simulink model "ControlledGrid"  (R2015b)
settings: Solver=ode1  StartTime=0.0  StopTime=10  FixedStep=Ts  RelTol=1e-3
InitFcn:
  | ControlInit();
values from neighbouring files (symbols this model uses):
  Fnom = 50    [ControlInit.m]
  Grid_F = Fnom    (= 50)    [ControlInit.m]
  Grid_V = 400e3    (= 400000)    [ControlInit.m]
  Rad2Deg = 180/pi    (= 57.2956455309)    [ControlInit.m]
libraries: powerlib x16, powerlib_meascontrol x3, simulink x2
settings Model: Creator=Emilio  LastModifiedBy=Emilio

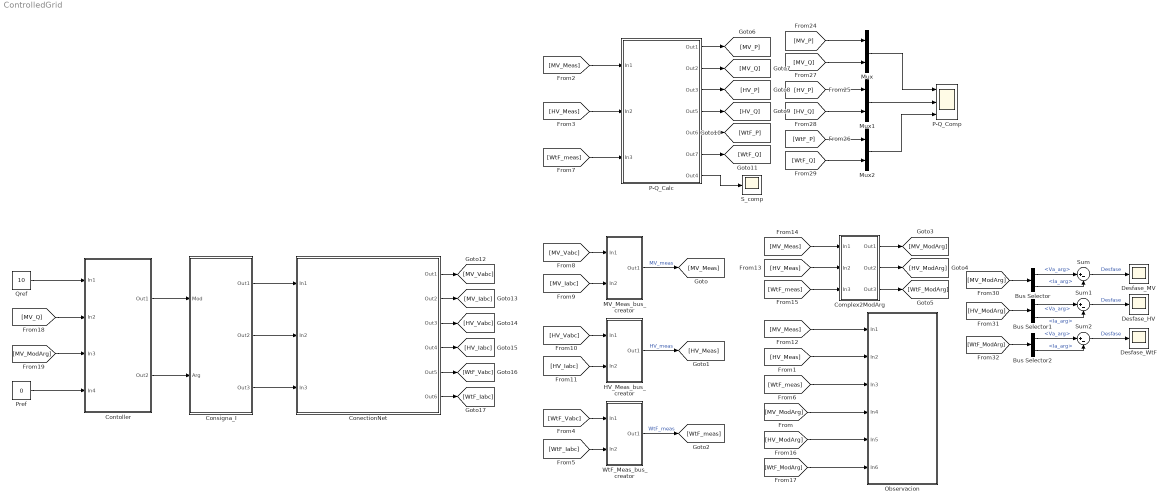
== system ControlledGrid ==
  Bus Selector : BusSelector  OutputSignals=V_ModArg.Va_arg,I_ModArg.Ia_arg
  Bus Selector1 : BusSelector  OutputSignals=V_ModArg.Va_arg,I_ModArg.Ia_arg
  Bus Selector2 : BusSelector  OutputSignals=V_ModArg.Va_arg,I_ModArg.Ia_arg
  Complex2ModArg : Subsystem
  ConectionNet : Subsystem
  Consigna_I : Subsystem
  Contoller : Subsystem
  Desfase_HV : Scope
  Desfase_MV : Scope
  Desfase_WtF : Scope
  HV_Meas_bus_creator : Subsystem
  MV_Meas_bus_creator : Subsystem
  Mux : Mux  Inputs=2
  Mux1 : Mux  Inputs=2
  Mux2 : Mux  Inputs=2
  Observacion : Subsystem
  P-Q_Calc : Subsystem
  P-Q_Comp : Scope  NumInputPorts=3
  Pref : Constant  Value=0
  Qref : Constant  Value=10
  S_comp : Scope
  Sum : Sum  Inputs=|+-
  Sum1 : Sum  Inputs=|+-
  Sum2 : Sum  Inputs=|+-
  WtF_Meas_bus_creator : Subsystem
  wires:
  [MV_Meas] -> P-Q_Calc/1(In1)
  [HV_Meas] -> P-Q_Calc/2(In2)
  P-Q_Calc/7(Out4) -> S_comp/1
  [MV_Vabc] -> MV_Meas_bus_creator/1(In1)
  [MV_Iabc] -> MV_Meas_bus_creator/2(In2)
  MV_Meas_bus_creator/1(Out1) -> [MV_Meas]  "MV_meas"
  [HV_Vabc] -> HV_Meas_bus_creator/1(In1)
  [HV_Iabc] -> HV_Meas_bus_creator/2(In2)
  HV_Meas_bus_creator/1(Out1) -> [HV_Meas]  "HV_meas"
  [WtF_Vabc] -> WtF_Meas_bus_creator/1(In1)
  [WtF_Iabc] -> WtF_Meas_bus_creator/2(In2)
  WtF_Meas_bus_creator/1(Out1) -> [WtF_meas]  "WtF_meas"
  [WtF_meas] -> P-Q_Calc/3(In3)
  [MV_Meas] -> Observacion/1(In1)
  [HV_Meas] -> Observacion/2(In2)
  [WtF_meas] -> Observacion/3(In3)
  [MV_ModArg] -> Observacion/4(In4)
  [HV_ModArg] -> Observacion/5(In5)
  [WtF_ModArg] -> Observacion/6(In6)
  P-Q_Calc/1(Out1) -> [MV_P]
  P-Q_Calc/2(Out2) -> [MV_Q]
  P-Q_Calc/3(Out3) -> [HV_P]
  P-Q_Calc/4(Out5) -> [HV_Q]
  P-Q_Calc/5(Out6) -> [WtF_P]
  P-Q_Calc/6(Out7) -> [WtF_Q]
  ConectionNet/1(Out1) -> [MV_Vabc]
  ConectionNet/2(Out2) -> [MV_Iabc]
  ConectionNet/3(Out3) -> [HV_Vabc]
  ConectionNet/4(Out4) -> [HV_Iabc]
  ConectionNet/5(Out5) -> [WtF_Vabc]
  ConectionNet/6(Out6) -> [WtF_Iabc]
  Consigna_I/1(Out1) -> ConectionNet/1(In1)
  Consigna_I/2(Out2) -> ConectionNet/2(In2)
  Consigna_I/3(Out3) -> ConectionNet/3(In3)
  [MV_Meas] -> Complex2ModArg/1(In1)
  [HV_Meas] -> Complex2ModArg/2(In2)
  [WtF_meas] -> Complex2ModArg/3(In3)
  Complex2ModArg/1(Out1) -> [MV_ModArg]
  Complex2ModArg/2(Out2) -> [HV_ModArg]
  Complex2ModArg/3(Out3) -> [WtF_ModArg]
  [MV_P] -> Mux/1
  [MV_Q] -> Mux/2
  [HV_Q] -> Mux1/2
  [HV_P] -> Mux1/1
  [WtF_P] -> Mux2/1
  [WtF_Q] -> Mux2/2
  Mux/1 -> P-Q_Comp/1
  Mux1/1 -> P-Q_Comp/2
  Mux2/1 -> P-Q_Comp/3
  [MV_ModArg] -> Bus Selector/1
  Bus Selector/1 -> Sum/1  "<Va_arg>"
  Bus Selector/2 -> Sum/2  "<Ia_arg>"
  Sum/1 -> Desfase_MV/1  "Desfase"
  [HV_ModArg] -> Bus Selector1/1
  Bus Selector1/1 -> Sum1/1  "<Va_arg>"
  Bus Selector1/2 -> Sum1/2  "<Ia_arg>"
  Sum1/1 -> Desfase_HV/1  "Desfase"
  Bus Selector2/1 -> Sum2/1  "<Va_arg>"
  Bus Selector2/2 -> Sum2/2  "<Ia_arg>"
  Sum2/1 -> Desfase_WtF/1  "Desfase"
  [WtF_ModArg] -> Bus Selector2/1
  Qref/1 -> Contoller/1(In1)
  [MV_Q] -> Contoller/2(In2)
  [MV_ModArg] -> Contoller/3(In3)
  Contoller/1(Out1) -> Consigna_I/1(Mod)
  Pref/1 -> Contoller/4(In4)
  Contoller/2(Out2) -> Consigna_I/2(Arg)

== system ControlledGrid/Complex2ModArg ==
  In1 : Inport
  In2 : Inport  Port=2
  In3 : Inport  Port=3
  Bus Creator1 : BusCreator  Inputs=2
  Bus Creator2 : BusCreator  Inputs=2
  Bus Creator3 : BusCreator  Inputs=2
  Bus Selector3 : BusSelector  OutputSignals=V_meas.Va,V_meas.Vb,V_meas.Vc,I_meas.Ia,I_meas.Ib,I_meas.Ic
  Bus Selector4 : BusSelector  OutputSignals=V_meas.Va,V_meas.Vb,V_meas.Vc,I_meas.Ia,I_meas.Ib,I_meas.Ic
  Bus Selector5 : BusSelector  OutputSignals=V_meas.Va,V_meas.Vb,V_meas.Vc,I_meas.Ia,I_meas.Ib,I_meas.Ic
  HV_mod&arg : Subsystem
  MV_mod&arg : Subsystem
  WtF_mod&arg : Subsystem
  Out1 : Outport
  Out2 : Outport  Port=2
  Out3 : Outport  Port=3
  wires:
  Bus Selector4/1 -> WtF_mod&arg/1(In1)  "<Va>"
  Bus Selector3/1 -> HV_mod&arg/1(In1)  "<Va>"
  Bus Selector3/2 -> HV_mod&arg/2(In2)  "<Vb>"
  Bus Selector3/3 -> HV_mod&arg/3(In3)  "<Vc>"
  Bus Selector3/4 -> HV_mod&arg/4(In4)  "<Ia>"
  Bus Selector3/6 -> HV_mod&arg/6(In6)  "<Ic>"
  HV_mod&arg/1(Out1) -> Bus Creator3/1
  In2/1 -> Bus Selector3/1
  HV_mod&arg/2(Out2) -> Bus Creator3/2
  In3/1 -> Bus Selector4/1
  Bus Selector3/5 -> HV_mod&arg/5(In5)  "<Ib>"
  Bus Selector4/6 -> WtF_mod&arg/6(In6)  "<Ic>"
  MV_mod&arg/1(Out1) -> Bus Creator2/1
  Bus Selector5/3 -> MV_mod&arg/3(In3)  "<Vc>"
  Bus Selector4/3 -> WtF_mod&arg/3(In3)  "<Vc>"
  Bus Selector4/2 -> WtF_mod&arg/2(In2)  "<Vb>"
  Bus Selector4/5 -> WtF_mod&arg/5(In5)  "<Ib>"
  Bus Creator3/1 -> Out2/1  "HV_ModArg"
  Bus Selector5/1 -> MV_mod&arg/1(In1)  "<Va>"
  Bus Selector5/6 -> MV_mod&arg/6(In6)  "<Ic>"
  Bus Selector5/5 -> MV_mod&arg/5(In5)  "<Ib>"
  Bus Creator2/1 -> Out1/1  "MV_ModArg"
  Bus Selector5/2 -> MV_mod&arg/2(In2)  "<Vb>"
  Bus Creator1/1 -> Out3/1  "WtF_ModArg"
  WtF_mod&arg/1(Out1) -> Bus Creator1/1
  WtF_mod&arg/2(Out2) -> Bus Creator1/2
  MV_mod&arg/2(Out2) -> Bus Creator2/2
  Bus Selector4/4 -> WtF_mod&arg/4(In4)  "<Ia>"
  Bus Selector5/4 -> MV_mod&arg/4(In4)  "<Ia>"
  In1/1 -> Bus Selector5/1

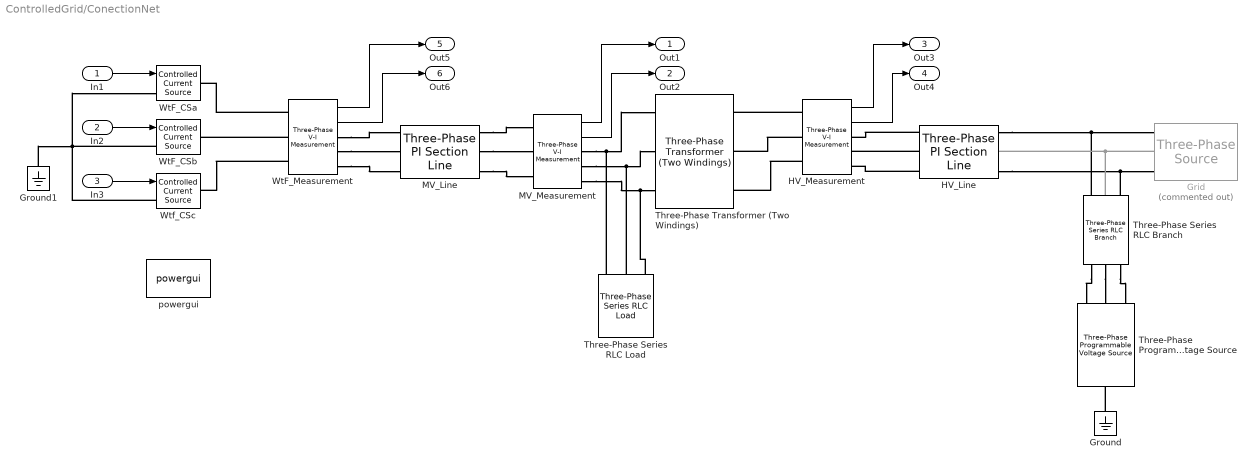
== system ControlledGrid/ConectionNet ==
  In1 : Inport
  In2 : Inport  Port=2
  In3 : Inport  Port=3
  Grid : powerlib/Electrical Sources/Three-Phase Source  Commented=on  InternalConnection=Yg  VoltagePhases=off  Voltage=Grid_V  PhaseAngle=0  Voltage_phases=[25e3 25e3 25e3]/sqrt(3)  PhaseAngles_phases=[0 -120 +120]  Frequency=Grid_F  NonIdealSource=on  SpecifyImpedance=off  Resistance=0.8929  Inductance=16.58e-3  ShortCircuitLevel=100e6  BaseVoltage=25e3  XRratio=7  BusType=PQ  Pref=10e3  Qref=0  Prefabc=[10e3, 10e3, 10e3]  Qrefabc=[0, 0, 0]  Qmin=-inf  Qmax=inf
  Ground : powerlib/Elements/Ground  LConnTagsString=a
  Ground1 : powerlib/Elements/Ground  LConnTagsString=a
  HV_Line : powerlib/Elements/Three-Phase PI Section Line  LConnTagsString=a|b|c  RConnTagsString=A|B|C  Frequency=50  Resistances=[ 0.01273 0.3864]  Inductances="[ 0.9337e-3  4.1264e-3]"  Capacitances=[12.74e-9 7.751e-9]  Length=100
  HV_Measurement : powerlib/Measurements/Three-Phase V-I Measurement  VoltageMeasurement=phase-to-ground  SetLabelV=off  LabelV=HV_Vabc  Vpu=off  VpuLL=off  CurrentMeasurement=yes  SetLabelI=off  LabelI=HV_Iabc  Ipu=off  Pbase=100e6  Vbase=500e3  OutputType=Complex  PhasorSimulation=on  PSBequivalent=0
  MV_Line : powerlib/Elements/Three-Phase PI Section Line  LConnTagsString=a|b|c  RConnTagsString=A|B|C  Frequency=50  Resistances=[ 0.01273 0.3864]  Inductances="[ 0.9337e-3  4.1264e-3]"  Capacitances="[ 0.9337e-3  4.1264e-3]"  Length=20
  MV_Measurement : powerlib/Measurements/Three-Phase V-I Measurement  VoltageMeasurement=phase-to-ground  SetLabelV=off  LabelV=MV_Vabc  Vpu=off  VpuLL=off  CurrentMeasurement=yes  SetLabelI=off  LabelI=MV_Iabc  Ipu=off  Pbase=100e6  Vbase=500e3  OutputType=Complex  PhasorSimulation=on  PSBequivalent=0
  Three-Phase Programmable Voltage Source : powerlib/Electrical Sources/Three-Phase Programmable Voltage Source  PositiveSequence="[Grid_V  0 Grid_F]"  VariationEntity=Amplitude  VariationType=Modulation  VariationTypeAlt=Step  VariationStep=0.5  VariationRate=10  VariationMagnitude=0  VariationFrequency=0.10  VariationTiming=[0 10]  VariationPhaseA=off  Amplitudes=[1 0.8 1.2 1.0]  TimeValues=[0 0.1 0.15 0.2]  HarmonicGeneration=off  HarmonicA=[3 0.2 -25 0]  HarmonicB=[2 0.15 35 2]  Timing="[0.05  3]"  BusType=PQ  Pref=0  Qref=0  Qmin=-inf  Qmax=inf
  Three-Phase Series RLC Branch : powerlib/Elements/Three-Phase Series RLC Branch  LConnTagsString=A|B|C  RConnTagsString=A|B|C  BranchType=RL  Resistance=1  Inductance=16.58e-3  Capacitance=0  Measurements=None
  Three-Phase Series RLC Load : powerlib/Elements/Three-Phase Series RLC Load  LConnTagsString=A|B|C  Configuration=Y (grounded)  NominalVoltage=1000  Vabc=[1e3 1e3 1e3]  Vabcp=[1e3 1e3 1e3]  NominalFrequency=60  UnbalancedPower=off  ActivePower=1  InductivePower=0  CapacitivePower=150e6  Pabc=[10e3 9e3 11e3]  QLabc=[100 90 110]  QCabc=[100 90 110]  Pabcp=[10e3 9e3 11e3]  QLabcp=[100 90 110]  QCabcp=[100 90 110]  Measurements=None  LoadType=constant Z
  Three-Phase Transformer (Two Windings) : powerlib/Elements/Three-Phase Transformer (Two Windings)  Winding1Connection=Yg  Winding2Connection=Yg  CoreType=Three single-phase transformers  SetSaturation=off  Hysteresis=off  DataFile='hysteresis'  SetInitialFlux=off  Measurements=None  UNITS=SI  NominalPower=[ 100e3 , 50 ]  Winding1=[22000 9.68 0.030812]  Winding2=[4e+05 3200 10.186]  Rm=2.42e+06  Lm=7703.1  L0=7.7033  Saturation=[0 0;0.0089072 68.613;3.7113 86.91]  InitialFluxes=[45.742 -45.742 40.024]  MoreParameters=off  BreakLoop=off  DataType=on  TransfoNumber=1
  WtF_CSa : powerlib/Electrical Sources/Controlled Current Source  Initialize=on  Source_Type=AC  Amplitude=12.9  Phase=0  Frequency=Fnom  Measurements=None
  WtF_CSb : powerlib/Electrical Sources/Controlled Current Source  Initialize=on  Source_Type=AC  Amplitude=12.9  Phase=120  Frequency=Fnom  Measurements=None
  WtF_Measurement : powerlib/Measurements/Three-Phase V-I Measurement  VoltageMeasurement=phase-to-ground  SetLabelV=off  LabelV=WtF_Vabc  Vpu=off  VpuLL=off  CurrentMeasurement=yes  SetLabelI=off  LabelI=WtF_Iabc  Ipu=off  Pbase=100e6  Vbase=500e3  OutputType=Complex  PhasorSimulation=on  PSBequivalent=0
  Wtf_CSc : powerlib/Electrical Sources/Controlled Current Source  Initialize=on  Source_Type=AC  Amplitude=12.9  Phase=-120  Frequency=Fnom  Measurements=None
  powergui : powerlib/powergui  Priority=1  SimulationMode=Phasor  SolverType=Tustin/Backward Euler (TBE)  SampleTime=50e-6  frequency=Fnom  SPID=off  DisableSnubberDevices=off  DisableRonSwitches=off  DisableVfSwitches=off  SwTol=0  DisplayEquations=off  Interpol=off  ExternalGateDelay=off  methode=off  Ts=10  FunctionMessages=off  echomessages=off  HookPort=off  EnableUseOfTLC=off  x0status=blocks  frequencyindice=50  Pbase=100e6  ErrMax=1e-4  Iterations=50  UnitsV=V  UnitsW=W  buscounter=0  RestoreLinks=warning  ResistiveCurrentMeasurement=off  Frange=[0:2:500]  Ylog=off  Xlog=on  ShowGrid=off  save=off  variable=ZData  structure=0  ZoomFFT=off  StartTime=0.0  cycles=1  DisplayStyle=1  fundamental=60  FreqAxis=off  MaxFrequency=1000  frequencyindicesteady=1  RmsSteady=1  display=off
  Out1 : Outport
  Out2 : Outport  Port=2
  Out3 : Outport  Port=3
  Out4 : Outport  Port=4
  Out5 : Outport  Port=5
  Out6 : Outport  Port=6
  wires:
  In1/1 -> WtF_CSa/1
  In2/1 -> WtF_CSb/1
  In3/1 -> Wtf_CSc/1
  MV_Measurement/1 -> Out1/1
  HV_Measurement/1 -> Out3/1
  HV_Measurement/2 -> Out4/1
  MV_Measurement/2 -> Out2/1
  WtF_Measurement/1 -> Out5/1
  WtF_Measurement/2 -> Out6/1
  connections:
  HV_Line/LConn2 -- HV_Measurement/RConn2
  HV_Measurement/LConn2 -- Three-Phase Transformer (Two Windings)/RConn2
  Three-Phase Series RLC Branch/LConn3 -- HV_Line/RConn3 -- Grid/RConn1
  HV_Line/RConn1 -- Three-Phase Series RLC Branch/LConn1 -- Grid/RConn3
  Grid/RConn2 -- Three-Phase Series RLC Branch/LConn2 -- HV_Line/RConn2
  HV_Measurement/LConn1 -- Three-Phase Transformer (Two Windings)/RConn1
  HV_Measurement/LConn3 -- Three-Phase Transformer (Two Windings)/RConn3
  MV_Measurement/RConn2 -- Three-Phase Series RLC Load/LConn2 -- Three-Phase Transformer (Two Windings)/LConn2
  MV_Measurement/RConn3 -- Three-Phase Series RLC Load/LConn3 -- Three-Phase Transformer (Two Windings)/LConn3
  MV_Measurement/RConn1 -- Three-Phase Transformer (Two Windings)/LConn1 -- Three-Phase Series RLC Load/LConn1
  HV_Line/LConn1 -- HV_Measurement/RConn1
  MV_Line/RConn1 -- MV_Measurement/LConn1
  MV_Line/RConn3 -- MV_Measurement/LConn3
  WtF_Measurement/LConn3 -- Wtf_CSc/RConn1
  WtF_Measurement/LConn1 -- WtF_CSa/RConn1
  MV_Line/RConn2 -- MV_Measurement/LConn2
  WtF_Measurement/LConn2 -- WtF_CSb/RConn1
  Ground/LConn1 -- Three-Phase Programmable Voltage Source/LConn1
  Three-Phase Series RLC Branch/RConn3 -- Three-Phase Programmable Voltage Source/RConn3
  Three-Phase Series RLC Branch/RConn1 -- Three-Phase Programmable Voltage Source/RConn1
  Three-Phase Series RLC Branch/RConn2 -- Three-Phase Programmable Voltage Source/RConn2
  WtF_Measurement/RConn3 -- MV_Line/LConn3
  WtF_Measurement/RConn2 -- MV_Line/LConn2
  WtF_Measurement/RConn1 -- MV_Line/LConn1
  HV_Line/LConn3 -- HV_Measurement/RConn3
  Wtf_CSc/LConn1 -- WtF_CSa/LConn1 -- Ground1/LConn1 -- WtF_CSb/LConn1

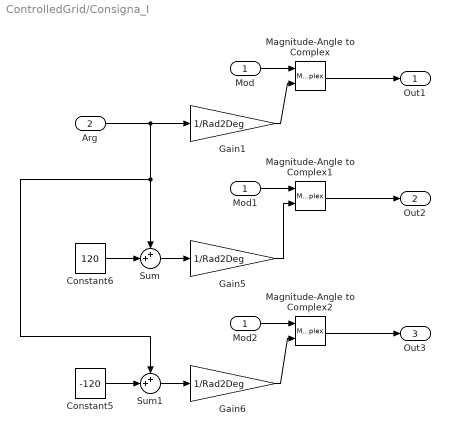
== system ControlledGrid/Consigna_I ==
  Mod : Inport
  Arg : Inport  Port=2
  Constant5 : Constant  Value=-120
  Constant6 : Constant  Value=120
  Gain1 : Gain  Gain=1/Rad2Deg
  Gain5 : Gain  Gain=1/Rad2Deg
  Gain6 : Gain  Gain=1/Rad2Deg
  Magnitude-Angle to Complex : MagnitudeAngleToComplex
  Magnitude-Angle to Complex1 : MagnitudeAngleToComplex
  Magnitude-Angle to Complex2 : MagnitudeAngleToComplex
  Mod1 : InportShadow
  Mod2 : InportShadow
  Sum : Sum  Inputs=++|
  Sum1 : Sum  Inputs=++|
  Out1 : Outport
  Out2 : Outport  Port=2
  Out3 : Outport  Port=3
  wires:
  Magnitude-Angle to Complex/1 -> Out1/1
  Magnitude-Angle to Complex1/1 -> Out2/1
  Magnitude-Angle to Complex2/1 -> Out3/1
  Gain5/1 -> Magnitude-Angle to Complex1/2
  Gain6/1 -> Magnitude-Angle to Complex2/2
  Mod2/1 -> Magnitude-Angle to Complex2/1
  Mod1/1 -> Magnitude-Angle to Complex1/1
  Mod/1 -> Magnitude-Angle to Complex/1
  Arg/1 -> Gain1/1, Sum/1, Sum1/1
  Sum1/1 -> Gain6/1
  Constant5/1 -> Sum1/2
  Sum/1 -> Gain5/1
  Constant6/1 -> Sum/2
  Gain1/1 -> Magnitude-Angle to Complex/2

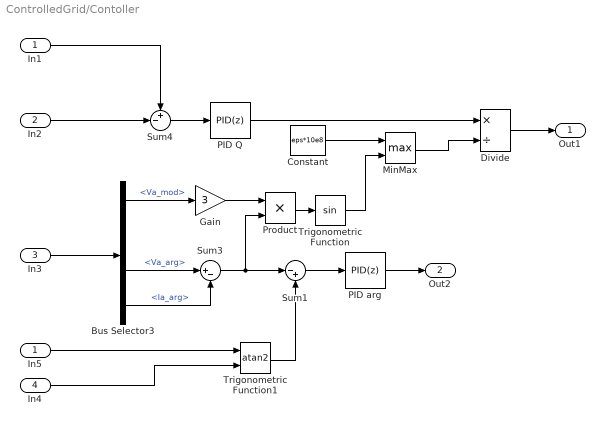
== system ControlledGrid/Contoller ==
  In1 : Inport
  In2 : Inport  Port=2
  In3 : Inport  Port=3
  In4 : Inport  Port=4
  " PID arg" : simulink/Continuous/PID Controller  Controller=PID  TimeDomain=Discrete-time  SampleTime=-1  IntegratorMethod=Forward Euler  FilterMethod=Forward Euler  Form=Parallel  UseFilter=on  ControllerParametersSource=internal  P=1  I=1  D=0  N=100  InitialConditionSource=internal  InitialConditionForIntegrator=0  InitialConditionForFilter=0  ExternalReset=none  LimitOutput=off  UpperSaturationLimit=inf  LowerSaturationLimit=-inf  LinearizeAsGain=off  AntiWindupMode=none  Kb=1  TrackingMode=off  Kt=1  PParamMin=[]  PParamMax=[]  IParamMin=[]  IParamMax=[]  DParamMin=[]  DParamMax=[]  NParamMin=[]  NParamMax=[]  KbParamMin=[]  KbParamMax=[]  KtParamMin=[]  KtParamMax=[]  POutMin=[]  POutMax=[]  IOutMin=[]  IOutMax=[]  DOutMin=[]  DOutMax=[]  NOutMin=[]  NOutMax=[]  KbOutMin=[]  KbOutMax=[]  KtOutMin=[]  KtOutMax=[]  IntegratorOutMin=[]  IntegratorOutMax=[]  FilterOutMin=[]  FilterOutMax=[]  SumOutMin=[]  SumOutMax=[]  SumI1OutMin=[]  SumI1OutMax=[]  SumI2OutMin=[]  SumI2OutMax=[]  SumI3OutMin=[]  SumI3OutMax=[]  SumDOutMin=[]  SumDOutMax=[]  SaturationOutMin=[]  SaturationOutMax=[]  IntegratorContinuousStateAttributes=''  IntegratorStateMustResolveToSignalObject=off  IntegratorRTWStateStorageClass=Auto  FilterContinuousStateAttributes=''  FilterStateMustResolveToSignalObject=off  FilterRTWStateStorageClass=Auto  DifferentiatorICPrevScaledInput=0  DifferentiatorOutMin=[]  DifferentiatorOutMax=[]
  Bus Selector3 : BusSelector  OutputSignals=V_ModArg.Va_mod,I_ModArg.Ia_mod,V_ModArg.Va_arg,I_ModArg.Ia_arg
  Constant : Constant  Value=eps*10e8  OutDataTypeStr=double
  Divide : Product  Inputs=*/
  Gain : Gain  Gain=3
  In5 : InportShadow
  MinMax : MinMax  Function=max  Inputs=2
  PID Q : simulink/Continuous/PID Controller  Controller=PID  TimeDomain=Discrete-time  SampleTime=-1  IntegratorMethod=Forward Euler  FilterMethod=Forward Euler  Form=Parallel  UseFilter=on  ControllerParametersSource=internal  P=1  I=1  D=0  N=100  InitialConditionSource=internal  InitialConditionForIntegrator=0  InitialConditionForFilter=0  ExternalReset=none  LimitOutput=off  UpperSaturationLimit=inf  LowerSaturationLimit=-inf  LinearizeAsGain=off  AntiWindupMode=none  Kb=1  TrackingMode=off  Kt=1  PParamMin=[]  PParamMax=[]  IParamMin=[]  IParamMax=[]  DParamMin=[]  DParamMax=[]  NParamMin=[]  NParamMax=[]  KbParamMin=[]  KbParamMax=[]  KtParamMin=[]  KtParamMax=[]  POutMin=[]  POutMax=[]  IOutMin=[]  IOutMax=[]  DOutMin=[]  DOutMax=[]  NOutMin=[]  NOutMax=[]  KbOutMin=[]  KbOutMax=[]  KtOutMin=[]  KtOutMax=[]  IntegratorOutMin=[]  IntegratorOutMax=[]  FilterOutMin=[]  FilterOutMax=[]  SumOutMin=[]  SumOutMax=[]  SumI1OutMin=[]  SumI1OutMax=[]  SumI2OutMin=[]  SumI2OutMax=[]  SumI3OutMin=[]  SumI3OutMax=[]  SumDOutMin=[]  SumDOutMax=[]  SaturationOutMin=[]  SaturationOutMax=[]  IntegratorContinuousStateAttributes=''  IntegratorStateMustResolveToSignalObject=off  IntegratorRTWStateStorageClass=Auto  FilterContinuousStateAttributes=''  FilterStateMustResolveToSignalObject=off  FilterRTWStateStorageClass=Auto  DifferentiatorICPrevScaledInput=0  DifferentiatorOutMin=[]  DifferentiatorOutMax=[]
  Product : Product
  Sum1 : Sum  Inputs=|-+
  Sum3 : Sum  Inputs=|+-
  Sum4 : Sum  Inputs=+-|
  Trigonometric Function : Trigonometry
  Trigonometric Function1 : Trigonometry  Operator=atan2
  Out1 : Outport
  Out2 : Outport  Port=2
  wires:
  Gain/1 -> Product/1
  Bus Selector3/4 -> Sum3/2  "<Ia_arg>"
  In3/1 -> Bus Selector3/1
  Sum3/1 -> Sum1/1, Product/2
  Bus Selector3/1 -> Gain/1  "<Va_mod>"
  Bus Selector3/3 -> Sum3/1  "<Va_arg>"
  In2/1 -> Sum4/2
  In1/1 -> Sum4/1
  Sum4/1 -> PID Q/1
  PID Q/1 -> Divide/1
  Divide/1 -> Out1/1
  Product/1 -> Trigonometric Function/1
  " PID arg"/1 -> Out2/1
  Sum1/1 -> " PID arg"/1
  In5/1 -> Trigonometric Function1/1
  In4/1 -> Trigonometric Function1/2
  Trigonometric Function1/1 -> Sum1/2
  MinMax/1 -> Divide/2
  Trigonometric Function/1 -> MinMax/2
  Constant/1 -> MinMax/1

== system ControlledGrid/HV_Meas_bus_creator ==
  In1 : Inport
  In2 : Inport  Port=2
  " " : ComplexToRealImag
  " 1" : ComplexToRealImag
  Bus Creator : BusCreator  Inputs=2
  Bus Creator1 : BusCreator  Inputs=6
  Bus Creator2 : BusCreator  Inputs=6
  Demux4 : Demux  Outputs=3
  Demux5 : Demux  Outputs=3
  Out1 : Outport  OutDataTypeStr=Bus: HV_meas
  wires:
  " "/1 -> Bus Creator2/3  "Ia_real"
  In1/1 -> Demux4/1, Bus Creator1/1  "Vabc"
  In2/1 -> Demux5/1, Bus Creator2/1  "Iabc"
  " 1"/2 -> Bus Creator1/4  "Va_img"
  Demux4/1 -> " 1"/1, Bus Creator1/2  "Va"
  Demux4/2 -> Bus Creator1/5  "Vb"
  Demux5/3 -> Bus Creator2/6  "Ic"
  " "/2 -> Bus Creator2/4  "Ia_img"
  Demux5/2 -> Bus Creator2/5  "Ib"
  Bus Creator/1 -> Out1/1
  " 1"/1 -> Bus Creator1/3  "Va_real"
  Demux5/1 -> Bus Creator2/2, " "/1  "Ia"
  Bus Creator2/1 -> Bus Creator/2  "I_meas"
  Bus Creator1/1 -> Bus Creator/1  "V_meas"
  Demux4/3 -> Bus Creator1/6  "Vc"

== system ControlledGrid/MV_Meas_bus_creator ==
  note: Creacion de los buses de medidas de los parametros de la red
  In1 : Inport
  In2 : Inport  Port=2
  " " : ComplexToRealImag
  "  " : ComplexToRealImag
  Bus Creator : BusCreator  Inputs=2
  Bus Creator1 : BusCreator  Inputs=6
  Bus Creator2 : BusCreator  Inputs=6
  Demux4 : Demux  Outputs=3
  Demux5 : Demux  Outputs=3
  Out1 : Outport  OutDataTypeStr=Bus: MV_meas
  wires:
  Demux4/3 -> Bus Creator1/6  "Vc"
  Bus Creator1/1 -> Bus Creator/1  "V_meas"
  Bus Creator2/1 -> Bus Creator/2  "I_meas"
  Demux5/1 -> " "/1, Bus Creator2/2  "Ia"
  "  "/1 -> Bus Creator1/3  "Va_real"
  Bus Creator/1 -> Out1/1
  Demux5/2 -> Bus Creator2/5  "Ib"
  " "/2 -> Bus Creator2/4  "Ia_img"
  Demux5/3 -> Bus Creator2/6  "Ic"
  Demux4/2 -> Bus Creator1/5  "Vb"
  Demux4/1 -> Bus Creator1/2, "  "/1  "Va"
  "  "/2 -> Bus Creator1/4  "Va_img"
  In2/1 -> Bus Creator2/1, Demux5/1  "Iabc"
  In1/1 -> Bus Creator1/1, Demux4/1  "Vabc"
  " "/1 -> Bus Creator2/3  "Ia_real"

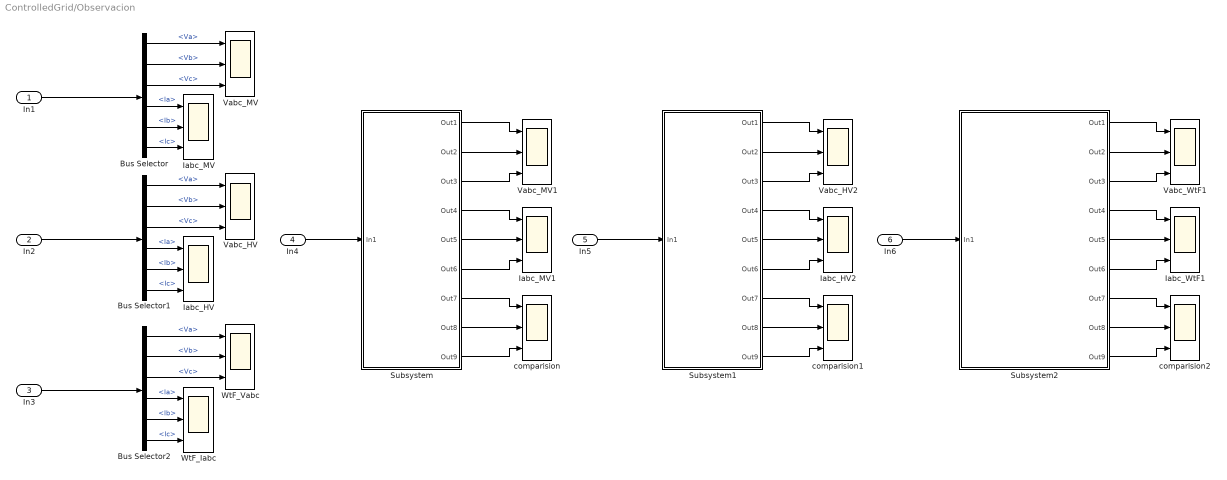
== system ControlledGrid/Observacion ==
  In1 : Inport  OutDataTypeStr=Bus: MV_meas
  In2 : Inport  Port=2  OutDataTypeStr=Bus: HV_meas
  In3 : Inport  Port=3  OutDataTypeStr=Bus: WtF_meas
  In4 : Inport  Port=4  OutDataTypeStr=Bus: MV_ModArg
  In5 : Inport  Port=5  OutDataTypeStr=Bus: HV_ModArg
  In6 : Inport  Port=6  OutDataTypeStr=Bus: WtF_ModArg
  Bus Selector : BusSelector  OutputSignals=V_meas.Va,V_meas.Vb,V_meas.Vc,I_meas.Ia,I_meas.Ib,I_meas.Ic
  Bus Selector1 : BusSelector  OutputSignals=V_meas.Va,V_meas.Vb,V_meas.Vc,I_meas.Ia,I_meas.Ib,I_meas.Ic
  Bus Selector2 : BusSelector  OutputSignals=V_meas.Va,V_meas.Vb,V_meas.Vc,I_meas.Ia,I_meas.Ib,I_meas.Ic
  Iabc_HV : Scope  NumInputPorts=3
  Iabc_HV2 : Scope  NumInputPorts=3
  Iabc_MV : Scope  NumInputPorts=3
  Iabc_MV1 : Scope  NumInputPorts=3
  Iabc_WtF1 : Scope  NumInputPorts=3
  Subsystem : Subsystem
  Subsystem1 : Subsystem
  Subsystem2 : Subsystem
  Vabc_HV : Scope  NumInputPorts=3
  Vabc_HV2 : Scope  NumInputPorts=3
  Vabc_MV : Scope  NumInputPorts=3
  Vabc_MV1 : Scope  NumInputPorts=3
  Vabc_WtF1 : Scope  NumInputPorts=3
  WtF_Iabc : Scope  NumInputPorts=3
  WtF_Vabc : Scope  NumInputPorts=3
  comparision : Scope  NumInputPorts=3
  comparision1 : Scope  NumInputPorts=3
  comparision2 : Scope  NumInputPorts=3
  wires:
  Bus Selector/6 -> Iabc_MV/3  "<Ic>"
  Bus Selector/3 -> Vabc_MV/3  "<Vc>"
  Bus Selector/1 -> Vabc_MV/1  "<Va>"
  Bus Selector/4 -> Iabc_MV/1  "<Ia>"
  Bus Selector/2 -> Vabc_MV/2  "<Vb>"
  Bus Selector/5 -> Iabc_MV/2  "<Ib>"
  Bus Selector1/1 -> Vabc_HV/1  "<Va>"
  Bus Selector1/4 -> Iabc_HV/1  "<Ia>"
  Bus Selector1/2 -> Vabc_HV/2  "<Vb>"
  Bus Selector2/1 -> WtF_Vabc/1  "<Va>"
  In1/1 -> Bus Selector/1
  In2/1 -> Bus Selector1/1
  Bus Selector2/2 -> WtF_Vabc/2  "<Vb>"
  Bus Selector1/6 -> Iabc_HV/3  "<Ic>"
  Bus Selector1/3 -> Vabc_HV/3  "<Vc>"
  In3/1 -> Bus Selector2/1
  Bus Selector1/5 -> Iabc_HV/2  "<Ib>"
  Bus Selector2/3 -> WtF_Vabc/3  "<Vc>"
  Bus Selector2/5 -> WtF_Iabc/2  "<Ib>"
  Bus Selector2/4 -> WtF_Iabc/1  "<Ia>"
  Bus Selector2/6 -> WtF_Iabc/3  "<Ic>"
  Subsystem1/1(Out1) -> Vabc_HV2/1
  Subsystem1/3(Out3) -> Vabc_HV2/3
  Subsystem1/5(Out5) -> Iabc_HV2/2
  Subsystem1/6(Out6) -> Iabc_HV2/3
  Subsystem1/8(Out8) -> comparision1/2
  Subsystem1/2(Out2) -> Vabc_HV2/2
  Subsystem1/7(Out7) -> comparision1/1
  Subsystem1/4(Out4) -> Iabc_HV2/1
  In5/1 -> Subsystem1/1(In1)
  Subsystem1/9(Out9) -> comparision1/3
  Subsystem/9(Out9) -> comparision/3
  Subsystem/8(Out8) -> comparision/2
  In4/1 -> Subsystem/1(In1)
  Subsystem/6(Out6) -> Iabc_MV1/3
  Subsystem/5(Out5) -> Iabc_MV1/2
  Subsystem/1(Out1) -> Vabc_MV1/1
  Subsystem/4(Out4) -> Iabc_MV1/1
  Subsystem/2(Out2) -> Vabc_MV1/2
  Subsystem/7(Out7) -> comparision/1
  Subsystem/3(Out3) -> Vabc_MV1/3
  In6/1 -> Subsystem2/1(In1)
  Subsystem2/2(Out2) -> Vabc_WtF1/2
  Subsystem2/3(Out3) -> Vabc_WtF1/3
  Subsystem2/1(Out1) -> Vabc_WtF1/1
  Subsystem2/4(Out4) -> Iabc_WtF1/1
  Subsystem2/5(Out5) -> Iabc_WtF1/2
  Subsystem2/6(Out6) -> Iabc_WtF1/3
  Subsystem2/7(Out7) -> comparision2/1
  Subsystem2/9(Out9) -> comparision2/3
  Subsystem2/8(Out8) -> comparision2/2

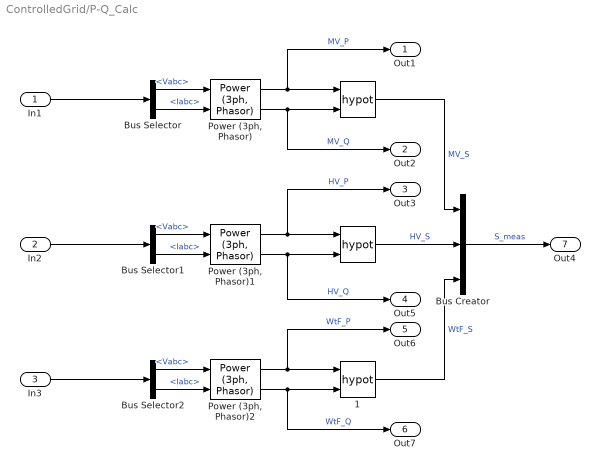
== system ControlledGrid/P-Q_Calc ==
  In1 : Inport  OutDataTypeStr=Bus: MV_meas
  In2 : Inport  Port=2  OutDataTypeStr=Bus: HV_meas
  In3 : Inport  Port=3  OutDataTypeStr=Bus: WtF_meas
  " " : Math  Operator=hypot  SaturateOnIntegerOverflow=on
  "  " : Math  Operator=hypot  SaturateOnIntegerOverflow=on
  "  1" : Math  Operator=hypot  SaturateOnIntegerOverflow=on
  Bus Creator : BusCreator  Inputs=3
  Bus Selector : BusSelector  OutputSignals=V_meas.Vabc,I_meas.Iabc
  Bus Selector1 : BusSelector  OutputSignals=V_meas.Vabc,I_meas.Iabc
  Bus Selector2 : BusSelector  OutputSignals=V_meas.Vabc,I_meas.Iabc
  "Power (3ph, Phasor)" : powerlib_meascontrol/Measurements/Power (3ph, Phasor)
  "Power (3ph, Phasor)1" : powerlib_meascontrol/Measurements/Power (3ph, Phasor)
  "Power (3ph, Phasor)2" : powerlib_meascontrol/Measurements/Power (3ph, Phasor)
  Out1 : Outport
  Out2 : Outport  Port=2
  Out3 : Outport  Port=3
  Out5 : Outport  Port=4
  Out6 : Outport  Port=5
  Out7 : Outport  Port=6
  Out4 : Outport  Port=7  OutDataTypeStr=Bus: S_meas
  wires:
  Bus Creator/1 -> Out4/1  "S_meas"
  "Power (3ph, Phasor)"/2 -> " "/2, Out2/1  "MV_Q"
  "Power (3ph, Phasor)1"/2 -> Out5/1, "  "/2  "HV_Q"
  " "/1 -> Bus Creator/1  "MV_S"
  "Power (3ph, Phasor)1"/1 -> Out3/1, "  "/1  "HV_P"
  "  "/1 -> Bus Creator/2  "HV_S"
  "Power (3ph, Phasor)"/1 -> " "/1, Out1/1  "MV_P"
  In1/1 -> Bus Selector/1
  Bus Selector/1 -> "Power (3ph, Phasor)"/1  "<Vabc>"
  Bus Selector/2 -> "Power (3ph, Phasor)"/2  "<Iabc>"
  In2/1 -> Bus Selector1/1
  Bus Selector1/1 -> "Power (3ph, Phasor)1"/1  "<Vabc>"
  Bus Selector1/2 -> "Power (3ph, Phasor)1"/2  "<Iabc>"
  "Power (3ph, Phasor)2"/2 -> "  1"/2, Out7/1  "WtF_Q"
  "Power (3ph, Phasor)2"/1 -> "  1"/1, Out6/1  "WtF_P"
  "  1"/1 -> Bus Creator/3  "WtF_S"
  In3/1 -> Bus Selector2/1
  Bus Selector2/1 -> "Power (3ph, Phasor)2"/1  "<Vabc>"
  Bus Selector2/2 -> "Power (3ph, Phasor)2"/2  "<Iabc>"

== system ControlledGrid/WtF_Meas_bus_creator ==
  In1 : Inport
  In2 : Inport  Port=2
  " " : ComplexToRealImag
  " 1" : ComplexToRealImag
  Bus Creator : BusCreator  Inputs=2
  Bus Creator1 : BusCreator  Inputs=6
  Bus Creator2 : BusCreator  Inputs=6
  Demux4 : Demux  Outputs=3
  Demux5 : Demux  Outputs=3
  Out1 : Outport  OutDataTypeStr=Bus: WtF_meas
  wires:
  Demux4/3 -> Bus Creator1/6  "Vc"
  Bus Creator1/1 -> Bus Creator/1  "V_meas"
  Bus Creator2/1 -> Bus Creator/2  "I_meas"
  Demux5/1 -> " "/1, Bus Creator2/2  "Ia"
  " 1"/1 -> Bus Creator1/3  "Va_real"
  Bus Creator/1 -> Out1/1
  Demux5/2 -> Bus Creator2/5  "Ib"
  " "/2 -> Bus Creator2/4  "Ia_img"
  Demux5/3 -> Bus Creator2/6  "Ic"
  Demux4/2 -> Bus Creator1/5  "Vb"
  Demux4/1 -> Bus Creator1/2, " 1"/1  "Va"
  " 1"/2 -> Bus Creator1/4  "Va_img"
  In2/1 -> Bus Creator2/1, Demux5/1  "Iabc"
  In1/1 -> Bus Creator1/1, Demux4/1  "Vabc"
  " "/1 -> Bus Creator2/3  "Ia_real"

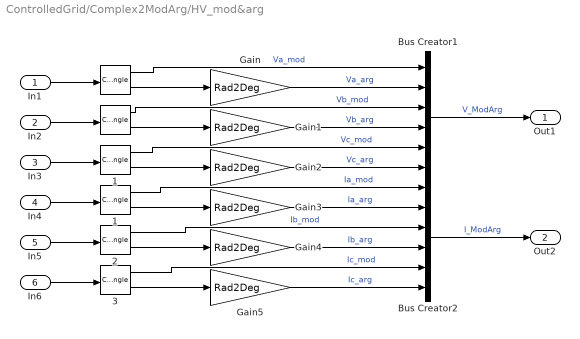
== system ControlledGrid/Complex2ModArg/HV_mod&arg ==
  In1 : Inport
  In2 : Inport  Port=2
  In3 : Inport  Port=3
  In4 : Inport  Port=4
  In5 : Inport  Port=5
  In6 : Inport  Port=6
  " " : ComplexToMagnitudeAngle
    {,1..3} (4 alike) : ComplexToMagnitudeAngle
  " 1" : ComplexToMagnitudeAngle
  Bus Creator1 : BusCreator  Inputs=6
  Bus Creator2 : BusCreator  Inputs=6
  Gain{,1..5} (6 alike) : Gain  Gain=Rad2Deg
  Out1 : Outport  OutDataTypeStr=Bus: V_ModArg
  Out2 : Outport  Port=2  OutDataTypeStr=Bus: I_ModArg
  wires:
  " "/2 -> Gain/1
  "  3"/2 -> Gain5/1
  " 1"/2 -> Gain3/1
  "  2"/1 -> Bus Creator2/3  "Ib_mod"
  " 1"/1 -> Bus Creator2/1  "Ia_mod"
  Gain2/1 -> Bus Creator1/6  "Vc_arg"
  "  1"/2 -> Gain2/1
  Gain1/1 -> Bus Creator1/4  "Vb_arg"
  Bus Creator1/1 -> Out1/1  "V_ModArg"
  "  "/2 -> Gain1/1
  "  "/1 -> Bus Creator1/3  "Vb_mod"
  "  2"/2 -> Gain4/1
  Gain/1 -> Bus Creator1/2  "Va_arg"
  Gain5/1 -> Bus Creator2/6  "Ic_arg"
  " "/1 -> Bus Creator1/1  "Va_mod"
  "  1"/1 -> Bus Creator1/5  "Vc_mod"
  Gain3/1 -> Bus Creator2/2  "Ia_arg"
  Bus Creator2/1 -> Out2/1  "I_ModArg"
  Gain4/1 -> Bus Creator2/4  "Ib_arg"
  "  3"/1 -> Bus Creator2/5  "Ic_mod"
  In5/1 -> "  2"/1
  In6/1 -> "  3"/1
  In4/1 -> " 1"/1
  In3/1 -> "  1"/1
  In2/1 -> "  "/1
  In1/1 -> " "/1

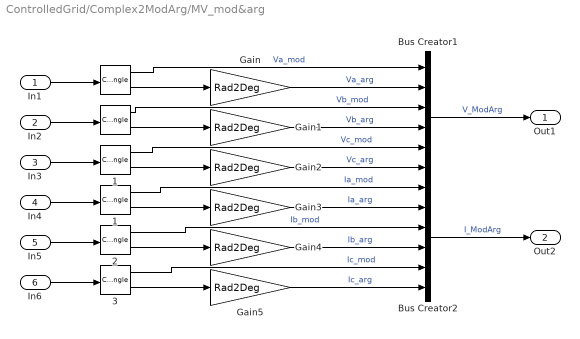
== system ControlledGrid/Complex2ModArg/MV_mod&arg ==
  In1 : Inport
  In2 : Inport  Port=2
  In3 : Inport  Port=3
  In4 : Inport  Port=4
  In5 : Inport  Port=5
  In6 : Inport  Port=6
  " " : ComplexToMagnitudeAngle
    {,1..3} (4 alike) : ComplexToMagnitudeAngle
  " 1" : ComplexToMagnitudeAngle
  Bus Creator1 : BusCreator  Inputs=6
  Bus Creator2 : BusCreator  Inputs=6
  Gain{,1..5} (6 alike) : Gain  Gain=Rad2Deg
  Out1 : Outport  OutDataTypeStr=Bus: V_ModArg
  Out2 : Outport  Port=2  OutDataTypeStr=Bus: I_ModArg
  wires:
  In1/1 -> " "/1
  In2/1 -> "  "/1
  In3/1 -> "  1"/1
  In4/1 -> " 1"/1
  In6/1 -> "  3"/1
  In5/1 -> "  2"/1
  "  3"/1 -> Bus Creator2/5  "Ic_mod"
  Gain4/1 -> Bus Creator2/4  "Ib_arg"
  Bus Creator2/1 -> Out2/1  "I_ModArg"
  Gain3/1 -> Bus Creator2/2  "Ia_arg"
  "  1"/1 -> Bus Creator1/5  "Vc_mod"
  " "/1 -> Bus Creator1/1  "Va_mod"
  Gain5/1 -> Bus Creator2/6  "Ic_arg"
  Gain/1 -> Bus Creator1/2  "Va_arg"
  "  2"/2 -> Gain4/1
  "  "/1 -> Bus Creator1/3  "Vb_mod"
  "  "/2 -> Gain1/1
  Bus Creator1/1 -> Out1/1  "V_ModArg"
  Gain1/1 -> Bus Creator1/4  "Vb_arg"
  "  1"/2 -> Gain2/1
  Gain2/1 -> Bus Creator1/6  "Vc_arg"
  " 1"/1 -> Bus Creator2/1  "Ia_mod"
  "  2"/1 -> Bus Creator2/3  "Ib_mod"
  " 1"/2 -> Gain3/1
  "  3"/2 -> Gain5/1
  " "/2 -> Gain/1

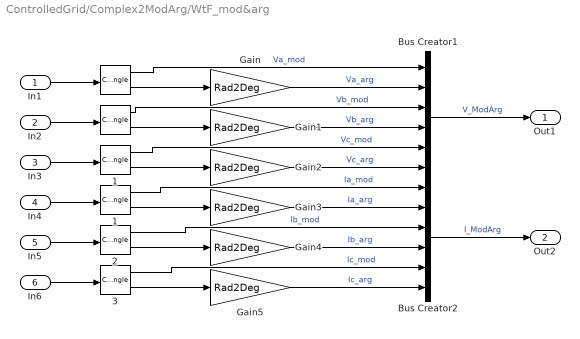
== system ControlledGrid/Complex2ModArg/WtF_mod&arg ==
  In1 : Inport
  In2 : Inport  Port=2
  In3 : Inport  Port=3
  In4 : Inport  Port=4
  In5 : Inport  Port=5
  In6 : Inport  Port=6
  " " : ComplexToMagnitudeAngle
    {,1..3} (4 alike) : ComplexToMagnitudeAngle
  " 1" : ComplexToMagnitudeAngle
  Bus Creator1 : BusCreator  Inputs=6
  Bus Creator2 : BusCreator  Inputs=6
  Gain{,1..5} (6 alike) : Gain  Gain=Rad2Deg
  Out1 : Outport  OutDataTypeStr=Bus: V_ModArg
  Out2 : Outport  Port=2  OutDataTypeStr=Bus: I_ModArg
  wires:
  In1/1 -> " "/1
  In2/1 -> "  "/1
  In3/1 -> "  1"/1
  In4/1 -> " 1"/1
  In6/1 -> "  3"/1
  In5/1 -> "  2"/1
  "  3"/1 -> Bus Creator2/5  "Ic_mod"
  Gain4/1 -> Bus Creator2/4  "Ib_arg"
  Bus Creator2/1 -> Out2/1  "I_ModArg"
  Gain3/1 -> Bus Creator2/2  "Ia_arg"
  "  1"/1 -> Bus Creator1/5  "Vc_mod"
  " "/1 -> Bus Creator1/1  "Va_mod"
  Gain5/1 -> Bus Creator2/6  "Ic_arg"
  Gain/1 -> Bus Creator1/2  "Va_arg"
  "  2"/2 -> Gain4/1
  "  "/1 -> Bus Creator1/3  "Vb_mod"
  "  "/2 -> Gain1/1
  Bus Creator1/1 -> Out1/1  "V_ModArg"
  Gain1/1 -> Bus Creator1/4  "Vb_arg"
  "  1"/2 -> Gain2/1
  Gain2/1 -> Bus Creator1/6  "Vc_arg"
  " 1"/1 -> Bus Creator2/1  "Ia_mod"
  "  2"/1 -> Bus Creator2/3  "Ib_mod"
  " 1"/2 -> Gain3/1
  "  3"/2 -> Gain5/1
  " "/2 -> Gain/1

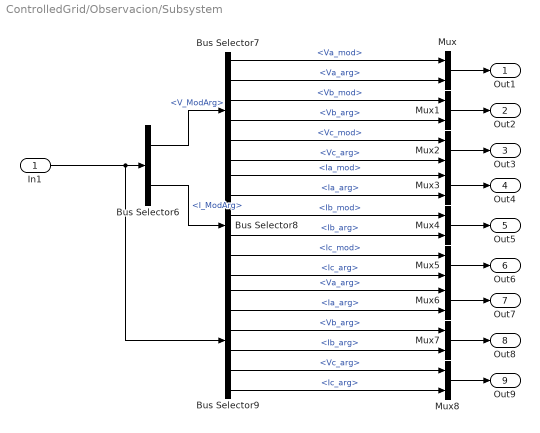
== system ControlledGrid/Observacion/Subsystem ==
  In1 : Inport  OutDataTypeStr=Bus: MV_ModArg
  Bus Selector6 : BusSelector  OutputSignals=V_ModArg,I_ModArg
  Bus Selector7 : BusSelector  OutputSignals=Va_mod,Va_arg,Vb_mod,Vb_arg,Vc_mod,Vc_arg
  Bus Selector8 : BusSelector  OutputSignals=Ia_mod,Ia_arg,Ib_mod,Ib_arg,Ic_mod,Ic_arg
  Bus Selector9 : BusSelector  OutputSignals=V_ModArg.Va_arg,I_ModArg.Ia_arg,V_ModArg.Vb_arg,I_ModArg.Ib_arg,V_ModArg.Vc_arg,I_ModArg.Ic_arg
  Mux{,1..8} (9 alike) : Mux  Inputs=2
  Out1 : Outport
  Out2 : Outport  Port=2
  Out3 : Outport  Port=3
  Out4 : Outport  Port=4
  Out5 : Outport  Port=5
  Out6 : Outport  Port=6
  Out7 : Outport  Port=7
  Out8 : Outport  Port=8
  Out9 : Outport  Port=9
  wires:
  Mux/1 -> Out1/1
  Bus Selector6/1 -> Bus Selector7/1  "<V_ModArg>"
  Bus Selector7/1 -> Mux/1  "<Va_mod>"
  Bus Selector9/4 -> Mux7/2  "<Ib_arg>"
  Mux6/1 -> Out7/1
  Mux7/1 -> Out8/1
  Bus Selector9/3 -> Mux7/1  "<Vb_arg>"
  Bus Selector9/6 -> Mux8/2  "<Ic_arg>"
  Bus Selector9/1 -> Mux6/1  "<Va_arg>"
  Bus Selector9/2 -> Mux6/2  "<Ia_arg>"
  Mux8/1 -> Out9/1
  Bus Selector9/5 -> Mux8/1  "<Vc_arg>"
  Bus Selector7/3 -> Mux1/1  "<Vb_mod>"
  Bus Selector7/5 -> Mux2/1  "<Vc_mod>"
  Bus Selector7/6 -> Mux2/2  "<Vc_arg>"
  Mux2/1 -> Out3/1
  Mux1/1 -> Out2/1
  Bus Selector7/2 -> Mux/2  "<Va_arg>"
  Bus Selector8/6 -> Mux5/2  "<Ic_arg>"
  Bus Selector8/4 -> Mux4/2  "<Ib_arg>"
  Bus Selector8/1 -> Mux3/1  "<Ia_mod>"
  Mux3/1 -> Out4/1
  Bus Selector8/5 -> Mux5/1  "<Ic_mod>"
  Mux4/1 -> Out5/1
  Bus Selector8/3 -> Mux4/1  "<Ib_mod>"
  Bus Selector8/2 -> Mux3/2  "<Ia_arg>"
  Mux5/1 -> Out6/1
  Bus Selector6/2 -> Bus Selector8/1  "<I_ModArg>"
  Bus Selector7/4 -> Mux1/2  "<Vb_arg>"
  In1/1 -> Bus Selector9/1, Bus Selector6/1

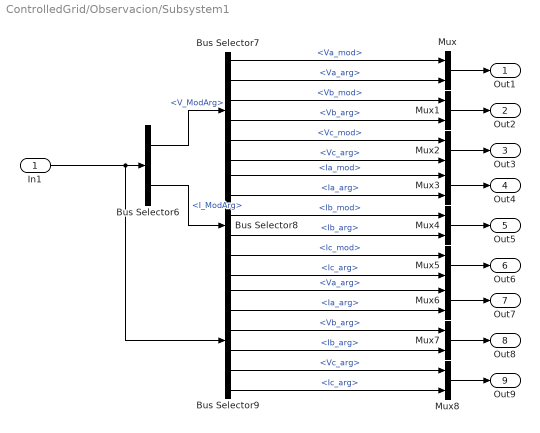
== system ControlledGrid/Observacion/Subsystem1 ==
  In1 : Inport  OutDataTypeStr=Bus: HV_ModArg
  Bus Selector6 : BusSelector  OutputSignals=V_ModArg,I_ModArg
  Bus Selector7 : BusSelector  OutputSignals=Va_mod,Va_arg,Vb_mod,Vb_arg,Vc_mod,Vc_arg
  Bus Selector8 : BusSelector  OutputSignals=Ia_mod,Ia_arg,Ib_mod,Ib_arg,Ic_mod,Ic_arg
  Bus Selector9 : BusSelector  OutputSignals=V_ModArg.Va_arg,I_ModArg.Ia_arg,V_ModArg.Vb_arg,I_ModArg.Ib_arg,V_ModArg.Vc_arg,I_ModArg.Ic_arg
  Mux{,1..8} (9 alike) : Mux  Inputs=2
  Out1 : Outport
  Out2 : Outport  Port=2
  Out3 : Outport  Port=3
  Out4 : Outport  Port=4
  Out5 : Outport  Port=5
  Out6 : Outport  Port=6
  Out7 : Outport  Port=7
  Out8 : Outport  Port=8
  Out9 : Outport  Port=9
  wires:
  In1/1 -> Bus Selector6/1, Bus Selector9/1
  Bus Selector7/4 -> Mux1/2  "<Vb_arg>"
  Bus Selector6/2 -> Bus Selector8/1  "<I_ModArg>"
  Mux5/1 -> Out6/1
  Bus Selector8/2 -> Mux3/2  "<Ia_arg>"
  Bus Selector8/3 -> Mux4/1  "<Ib_mod>"
  Mux4/1 -> Out5/1
  Bus Selector8/5 -> Mux5/1  "<Ic_mod>"
  Mux3/1 -> Out4/1
  Bus Selector8/1 -> Mux3/1  "<Ia_mod>"
  Bus Selector8/4 -> Mux4/2  "<Ib_arg>"
  Bus Selector8/6 -> Mux5/2  "<Ic_arg>"
  Bus Selector7/2 -> Mux/2  "<Va_arg>"
  Mux1/1 -> Out2/1
  Mux2/1 -> Out3/1
  Bus Selector7/6 -> Mux2/2  "<Vc_arg>"
  Bus Selector7/5 -> Mux2/1  "<Vc_mod>"
  Bus Selector7/3 -> Mux1/1  "<Vb_mod>"
  Bus Selector9/5 -> Mux8/1  "<Vc_arg>"
  Mux8/1 -> Out9/1
  Bus Selector9/2 -> Mux6/2  "<Ia_arg>"
  Bus Selector9/1 -> Mux6/1  "<Va_arg>"
  Bus Selector9/6 -> Mux8/2  "<Ic_arg>"
  Bus Selector9/3 -> Mux7/1  "<Vb_arg>"
  Mux7/1 -> Out8/1
  Mux6/1 -> Out7/1
  Bus Selector9/4 -> Mux7/2  "<Ib_arg>"
  Bus Selector7/1 -> Mux/1  "<Va_mod>"
  Bus Selector6/1 -> Bus Selector7/1  "<V_ModArg>"
  Mux/1 -> Out1/1

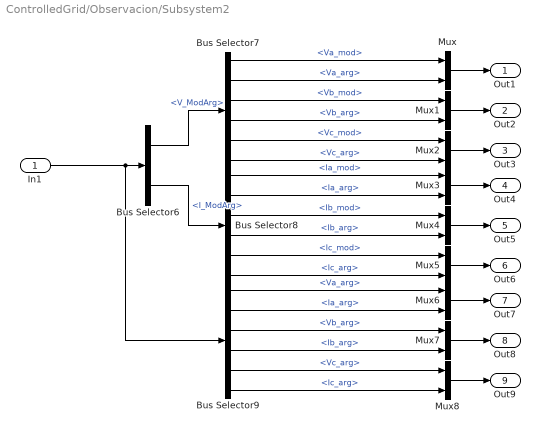
== system ControlledGrid/Observacion/Subsystem2 ==
  In1 : Inport  OutDataTypeStr=Bus: WtF_ModArg
  Bus Selector6 : BusSelector  OutputSignals=V_ModArg,I_ModArg
  Bus Selector7 : BusSelector  OutputSignals=Va_mod,Va_arg,Vb_mod,Vb_arg,Vc_mod,Vc_arg
  Bus Selector8 : BusSelector  OutputSignals=Ia_mod,Ia_arg,Ib_mod,Ib_arg,Ic_mod,Ic_arg
  Bus Selector9 : BusSelector  OutputSignals=V_ModArg.Va_arg,I_ModArg.Ia_arg,V_ModArg.Vb_arg,I_ModArg.Ib_arg,V_ModArg.Vc_arg,I_ModArg.Ic_arg
  Mux{,1..8} (9 alike) : Mux  Inputs=2
  Out1 : Outport
  Out2 : Outport  Port=2
  Out3 : Outport  Port=3
  Out4 : Outport  Port=4
  Out5 : Outport  Port=5
  Out6 : Outport  Port=6
  Out7 : Outport  Port=7
  Out8 : Outport  Port=8
  Out9 : Outport  Port=9
  wires:
  Mux/1 -> Out1/1
  Bus Selector6/1 -> Bus Selector7/1  "<V_ModArg>"
  Bus Selector7/1 -> Mux/1  "<Va_mod>"
  Bus Selector9/4 -> Mux7/2  "<Ib_arg>"
  Mux6/1 -> Out7/1
  Mux7/1 -> Out8/1
  Bus Selector9/3 -> Mux7/1  "<Vb_arg>"
  Bus Selector9/6 -> Mux8/2  "<Ic_arg>"
  Bus Selector9/1 -> Mux6/1  "<Va_arg>"
  Bus Selector9/2 -> Mux6/2  "<Ia_arg>"
  Mux8/1 -> Out9/1
  Bus Selector9/5 -> Mux8/1  "<Vc_arg>"
  Bus Selector7/3 -> Mux1/1  "<Vb_mod>"
  Bus Selector7/5 -> Mux2/1  "<Vc_mod>"
  Bus Selector7/6 -> Mux2/2  "<Vc_arg>"
  Mux2/1 -> Out3/1
  Mux1/1 -> Out2/1
  Bus Selector7/2 -> Mux/2  "<Va_arg>"
  Bus Selector8/6 -> Mux5/2  "<Ic_arg>"
  Bus Selector8/4 -> Mux4/2  "<Ib_arg>"
  Bus Selector8/1 -> Mux3/1  "<Ia_mod>"
  Mux3/1 -> Out4/1
  Bus Selector8/5 -> Mux5/1  "<Ic_mod>"
  Mux4/1 -> Out5/1
  Bus Selector8/3 -> Mux4/1  "<Ib_mod>"
  Bus Selector8/2 -> Mux3/2  "<Ia_arg>"
  Mux5/1 -> Out6/1
  Bus Selector6/2 -> Bus Selector8/1  "<I_ModArg>"
  Bus Selector7/4 -> Mux1/2  "<Vb_arg>"
  In1/1 -> Bus Selector9/1, Bus Selector6/1
